simulink model "ip"  (R2022b)
settings: Solver=FixedStepAuto  StartTime=0.0  StopTime=inf  FixedStep=Ts  RelTol=1e-3
values from neighbouring files (symbols this model uses):
  kLqr = [-58.3388321167 -3.68890430291 -0.316227766017 -0.543428779836 0.0629976019045]    [K_lqr.mat]    (also in calculate_lqr.m = lqr(A, B, Q, RLQR))
undefined symbols (not defined in the file or in its folder): countsPerRev, currentGain, currentOffset, motorN, pendDwnValue
libraries: arduinolib x6, arduinosensorlib x1, hdlsllib x1
settings Model: SimulationMode=external  ExtModeTrigDuration=2  Creator=47954  LastModifiedBy=47954
settings SolverCC: AutoInsertRateTranBlk=on
settings OptimizationCC: EnhancedBackFolding=on  PassReuseOutputArgsThreshold=0  MaxStackSize=64  OptimizeBlockOrder=speed  DifferentSizesBufferReuse=on  OptimizationCustomize=off
settings DebuggingCC: ParameterPrecisionLossMsg=none  ParameterTunabilityLossMsg=error
settings HardwareCC: ProdBitPerInt=16  ProdBitPerPointer=16  ProdBitPerSizeT=16  ProdBitPerPtrDiffT=16  ProdLargestAtomicFloat=None  ProdWordSize=8  ProdLongLongMode=on  ProdHWDeviceType=Atmel->AVR  UseEmbeddedCoderFeatures=off  UseSimulinkCoderFeatures=off
settings ModelReferenceCC: EnableRefExpFcnMdlSchedulingChecks=on
settings SFSimCC: MATLABDynamicMemAlloc=off
settings RTWCC: Description=Embedded Coder  SystemTargetFile=ert.tlc  HardwareBoard=Arduino Mega 2560  TemplateMakefile=ert_default_tmf  RTWVerbose=off  Toolchain=Arduino AVR
settings CodeAppCC: ForceParamTrailComments=on  OperatorAnnotations=on  MangleLength=10
settings ERTTargetCC: ERTCustomFileBanners=off  SupportContinuousTime=on  SupportNonInlinedSFcns=on  RemoveResetFunc=off  SupportVariableSizeSignals=on  ModelStepFunctionPrototypeControlCompliant=off  ExtMode=on  ExtModeTransport=3  ExtModeStaticAlloc=on  ExtModeStaticAllocSize=2048  ExtModeMexFile=ext_xcp  ExtModeMexArgs=0 6 921600  ExtModeIntrfLevel=Level2 - Open  ERTSrcFileBannerTemplate=codertarget_code_template.cgt  ERTHdrFileBannerTemplate=codertarget_code_template.cgt  ERTDataSrcFileTemplate=codertarget_code_template.cgt  ERTDataHdrFileTemplate=codertarget_code_template.cgt

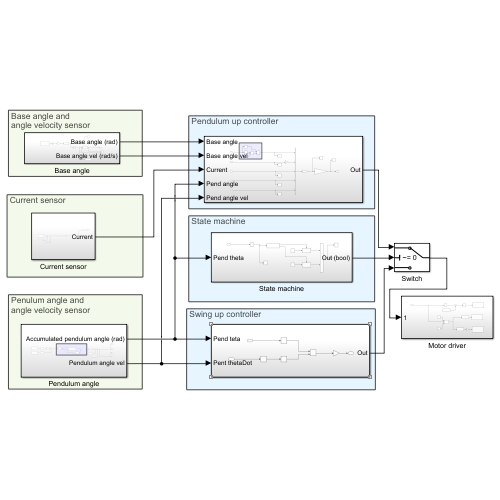
[thumbnail: Simulink's stored preview of the top-level diagram]
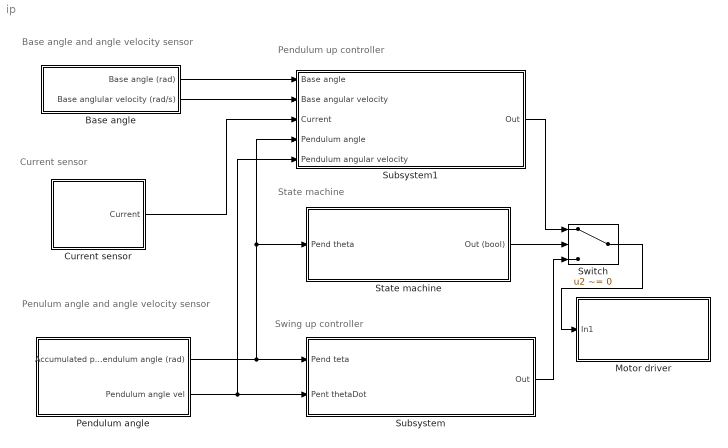
== system ip ==
  note: State machine
  note: Swing up controller
  note: Penulum angle and
      | angle velocity sensor
  note: Base angle and
      | angle velocity sensor
  note: Current sensor
  note: Pendulum up controller
  Base angle : Subsystem
  Current sensor : Subsystem
  Motor driver : Subsystem
  Pendulum angle : Subsystem
  State machine : Subsystem
  Subsystem : Subsystem
  Subsystem1 : Subsystem
  Switch : Switch  Criteria=u2 ~= 0  SaturateOnIntegerOverflow=off  InputSameDT=off
  wires:
  Pendulum angle/1(Accumulated pendulum angle (rad)) -> Subsystem1/4(Pendulum angle), State machine/1(Pend theta), Subsystem/1(Pend teta)
  State machine/1(Out (bool)) -> Switch/2
  Subsystem/1(Out) -> Switch/3
  Pendulum angle/2(Pendulum angle vel) -> Subsystem/2(Pent thetaDot), Subsystem1/5(Pendulum angular velocity)
  Subsystem1/1(Out) -> Switch/1
  Base angle/1(Base angle (rad)) -> Subsystem1/1(Base angle)
  Base angle/2(Base anglular velocity (rad/s)) -> Subsystem1/2(Base angular velocity)
  Switch/1 -> Motor driver/1(In1)
  Current sensor/1(Current) -> Subsystem1/3(Current)

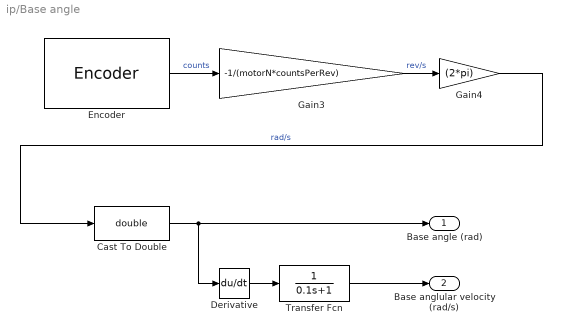
== system ip/Base angle ==
  Cast To Double : DataTypeConversion  OutDataTypeStr=double  SaturateOnIntegerOverflow=off  RndMeth=Floor
  Derivative : Derivative
  Encoder : arduinosensorlib/Encoder  InputA=2  InputB=3  Mode=No reset  SampleTime=-1
  Gain3 : Gain  Gain=-1/(motorN*countsPerRev)
  Gain4 : Gain  Gain=(2*pi)
  Transfer Fcn : TransferFcn  Denominator=[0.1 1]
  Base angle (rad) : Outport
  Base anglular velocity (rad/s) : Outport  Port=2
  wires:
  Gain3/1 -> Gain4/1  "rev/s"
  Gain4/1 -> Cast To Double/1  "rad/s"
  Encoder/1 -> Gain3/1  "counts"
  Transfer Fcn/1 -> Base anglular velocity (rad/s)/1
  Derivative/1 -> Transfer Fcn/1
  Cast To Double/1 -> Base angle (rad)/1, Derivative/1

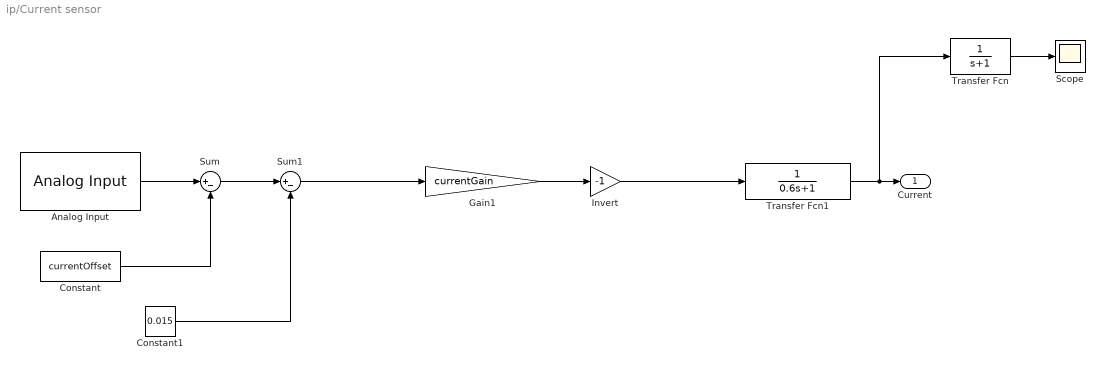
== system ip/Current sensor ==
  Analog Input : arduinolib/Analog Input  pinNumber=10  ReadResultsOnly=off  ConversionTriggerSource=Software  ExternalTriggerType=uint32( 0 )  OutputDataType=uint16  EnableConversionCompleteNotify=off  EnableOuputStatus=off  SampleTime=-1  blockPlatform=arduino
  Constant : Constant  Value=currentOffset
  Constant1 : Constant  Value=0.015
  Gain1 : Gain  Gain=currentGain
  Invert : Gain  Gain=-1
  Scope : Scope
  Sum : Sum  Inputs=|+-
  Sum1 : Sum  Inputs=|+-
  Transfer Fcn : TransferFcn  Denominator=[1 1]
  Transfer Fcn1 : TransferFcn  Denominator=[0.6 1]
  Current : Outport
  wires:
  Constant/1 -> Sum/2
  Analog Input/1 -> Sum/1
  Invert/1 -> Transfer Fcn1/1
  Sum/1 -> Sum1/1
  Gain1/1 -> Invert/1
  Transfer Fcn1/1 -> Transfer Fcn/1, Current/1
  Transfer Fcn/1 -> Scope/1
  Sum1/1 -> Gain1/1
  Constant1/1 -> Sum1/2

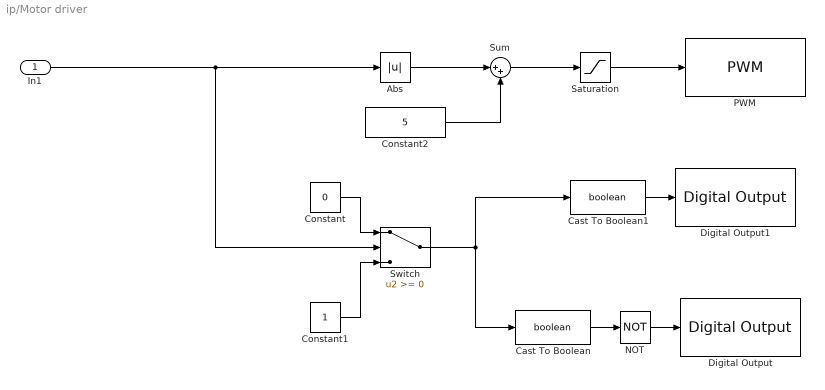
== system ip/Motor driver ==
  In1 : Inport
  Abs : Abs  SaturateOnIntegerOverflow=off
  Cast To Boolean : DataTypeConversion  OutDataTypeStr=boolean  SaturateOnIntegerOverflow=off  RndMeth=Floor
  Cast To Boolean1 : DataTypeConversion  OutDataTypeStr=boolean  SaturateOnIntegerOverflow=off  RndMeth=Floor
  Constant : Constant  Value=0
  Constant1 : Constant
  Constant2 : Constant  Value=5
  Digital Output : arduinolib/Digital Output  pinNumber=4  Direction=output  blockPlatform=arduino
  Digital Output1 : arduinolib/Digital Output  pinNumber=5  Direction=output  blockPlatform=arduino
  NOT : Logic  Operator=NOT  IconShape=distinctive  AllPortsSameDT=off  OutDataTypeStr=boolean
  PWM : arduinolib/PWM  pinNumber=13  frequencyType=Specify  desiredFrequency=490.2*2  achievableFrequency=980.4
  Saturation : Saturate  UpperLimit=255  LowerLimit=-255
  Sum : Sum  Inputs=|++
  Switch : Switch  SaturateOnIntegerOverflow=off  InputSameDT=off
  wires:
  Constant1/1 -> Switch/3
  Cast To Boolean1/1 -> Digital Output1/1
  Constant/1 -> Switch/1
  Constant2/1 -> Sum/2
  In1/1 -> Abs/1, Switch/2
  Switch/1 -> Cast To Boolean/1, Cast To Boolean1/1
  Cast To Boolean/1 -> NOT/1
  NOT/1 -> Digital Output/1
  Abs/1 -> Sum/1
  Sum/1 -> Saturation/1
  Saturation/1 -> PWM/1

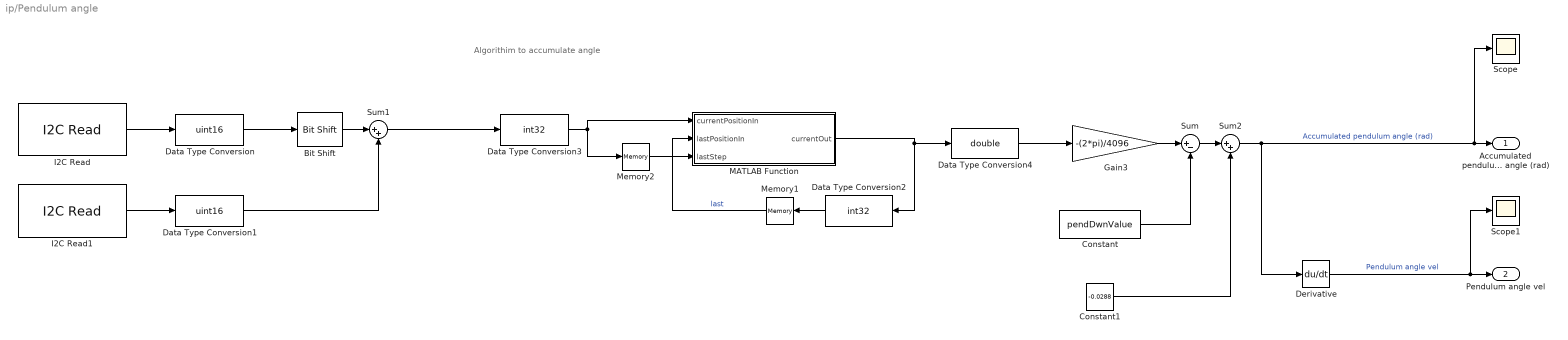
== system ip/Pendulum angle ==
  note: Algorithim to accumulate angle
  Bit Shift : hdlsllib/Logic and Bit Operations/Bit Shift  mode=Shift Left Logical  N=8
  Constant : Constant  Value=pendDwnValue
  Constant1 : Constant  Value=-0.0288
  Data Type Conversion : DataTypeConversion  OutDataTypeStr=uint16  SaturateOnIntegerOverflow=off  RndMeth=Floor
  Data Type Conversion1 : DataTypeConversion  OutDataTypeStr=uint16  SaturateOnIntegerOverflow=off  RndMeth=Floor
  Data Type Conversion2 : DataTypeConversion  OutDataTypeStr=int32  SaturateOnIntegerOverflow=off  RndMeth=Floor
  Data Type Conversion3 : DataTypeConversion  OutDataTypeStr=int32  SaturateOnIntegerOverflow=off  RndMeth=Floor
  Data Type Conversion4 : DataTypeConversion  OutDataTypeStr=double  SaturateOnIntegerOverflow=off  RndMeth=Floor
  Derivative : Derivative
  Gain3 : Gain  Gain=-(2*pi)/4096
  I2C Read : arduinolib/I2C Read  I2CModule=0  Mode=Master  SlaveAddress=0x36  SlaveByteOrder=BigEndian  Direction=Receiver  RegisterAddressMode=on  RegisterAddress=0x0c  SlaveDataType=uint8  DataLength=1  NoAck=off  RepeatedStart=off  OutputStatus=off  blockPlatform=ARDUINO  SampleTime=-1
  I2C Read1 : arduinolib/I2C Read  I2CModule=0  Mode=Master  SlaveAddress=0x36  SlaveByteOrder=BigEndian  Direction=Receiver  RegisterAddressMode=on  RegisterAddress=0x0d  SlaveDataType=uint8  DataLength=1  NoAck=off  RepeatedStart=off  OutputStatus=off  blockPlatform=ARDUINO  SampleTime=-1
  MATLAB Function : MATLAB Function  TreatAsAtomicUnit=on
  Memory1 : Memory
  Memory2 : Memory
  Scope : Scope
  Scope1 : Scope
  Sum : Sum  Inputs=|+-
  Sum1 : Sum  Inputs=|++
  Sum2 : Sum  Inputs=|++
  Accumulated pendulum angle (rad) : Outport
  Pendulum angle vel : Outport  Port=2
  wires:
  Memory2/1 -> MATLAB Function/3(lastStep)
  I2C Read/1 -> Data Type Conversion/1
  Data Type Conversion3/1 -> Memory2/1, MATLAB Function/1(currentPositionIn)
  Sum1/1 -> Data Type Conversion3/1
  I2C Read1/1 -> Data Type Conversion1/1
  Bit Shift/1 -> Sum1/1
  Memory1/1 -> MATLAB Function/2(lastPositionIn)  "last"
  Data Type Conversion1/1 -> Sum1/2
  Data Type Conversion/1 -> Bit Shift/1
  MATLAB Function/1(currentOut) -> Data Type Conversion2/1, Data Type Conversion4/1
  Data Type Conversion2/1 -> Memory1/1
  Data Type Conversion4/1 -> Gain3/1
  Gain3/1 -> Sum/1
  Constant/1 -> Sum/2
  Sum2/1 -> Accumulated pendulum angle (rad)/1, Scope/1, Derivative/1  "Accumulated pendulum angle (rad)"
  Sum/1 -> Sum2/1
  Constant1/1 -> Sum2/2
  Derivative/1 -> Scope1/1, Pendulum angle vel/1  "Pendulum angle vel"

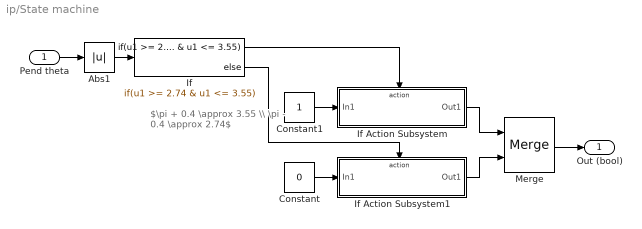
== system ip/State machine ==
  note: $\pi + 0.4 \approx 3.55 \\ \pi - 0.4 \approx 2.74$
  Pend theta : Inport
  Abs1 : Abs  SaturateOnIntegerOverflow=off
  Constant : Constant  Value=0
  Constant1 : Constant
  If : If  IfExpression=u1 >= 2.74 & u1 <= 3.55
  If Action Subsystem : Subsystem  TreatAsAtomicUnit=on
  If Action Subsystem1 : Subsystem  TreatAsAtomicUnit=on
  Merge : Merge
  Out (bool) : Outport
  wires:
  Constant1/1 -> If Action Subsystem/1(In1)
  If Action Subsystem/1(Out1) -> Merge/1
  If/1 -> If Action Subsystem/Action
  Pend theta/1 -> Abs1/1
  Merge/1 -> Out (bool)/1
  If/2 -> If Action Subsystem1/Action
  If Action Subsystem1/1(Out1) -> Merge/2
  Constant/1 -> If Action Subsystem1/1(In1)
  Abs1/1 -> If/1

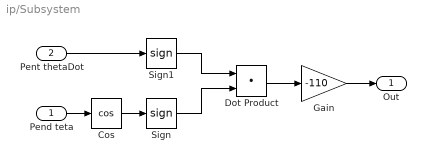
== system ip/Subsystem ==
  Pend teta : Inport
  Pent thetaDot : Inport  Port=2
  Cos : Trigonometry  Operator=cos
  Dot Product : DotProduct  OutDataTypeStr=Inherit: Inherit via internal rule
  Gain : Gain  Gain=-110
  Sign : Signum
  Sign1 : Signum
  Out : Outport
  wires:
  Pend teta/1 -> Cos/1
  Sign1/1 -> Dot Product/1
  Pent thetaDot/1 -> Sign1/1
  Dot Product/1 -> Gain/1
  Sign/1 -> Dot Product/2
  Cos/1 -> Sign/1
  Gain/1 -> Out/1

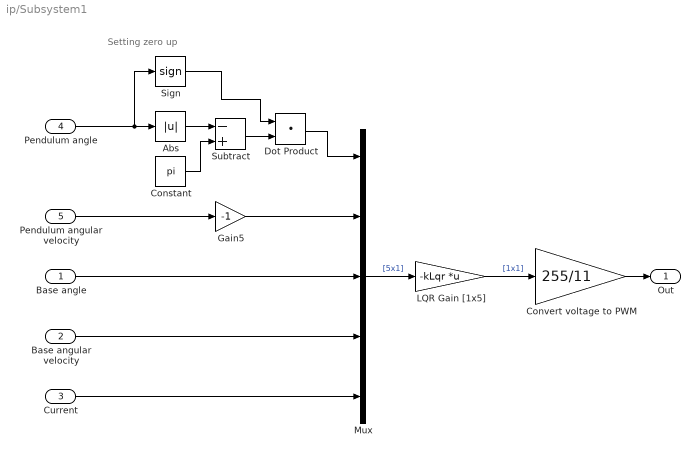
== system ip/Subsystem1 ==
  note: Setting zero up
  Base angle : Inport
  Base angular velocity : Inport  Port=2
  Current : Inport  Port=3
  Pendulum angle : Inport  Port=4
  Pendulum angular velocity : Inport  Port=5
  Abs : Abs  SaturateOnIntegerOverflow=off
  Constant : Constant  Value=pi
  Convert voltage to PWM : Gain  Gain=255/11
  Dot Product : DotProduct  OutDataTypeStr=Inherit: Inherit via internal rule
  Gain5 : Gain  Gain=-1
  LQR Gain [1x5] : Gain  Gain=-kLqr  Multiplication=Matrix(K*u)
  Mux : Mux  Inputs=5
  Sign : Signum
  Subtract : Sum  Inputs=-+
  Out : Outport
  wires:
  Pendulum angle/1 -> Sign/1, Abs/1
  Abs/1 -> Subtract/1
  Constant/1 -> Subtract/2
  Subtract/1 -> Dot Product/2
  Sign/1 -> Dot Product/1
  Dot Product/1 -> Mux/1
  Pendulum angular velocity/1 -> Gain5/1
  Base angle/1 -> Mux/3
  Base angular velocity/1 -> Mux/4
  Current/1 -> Mux/5
  Mux/1 -> LQR Gain [1x5]/1  "[5x1]"
  LQR Gain [1x5]/1 -> Convert voltage to PWM/1  "[1x1]"
  Convert voltage to PWM/1 -> Out/1
  Gain5/1 -> Mux/2

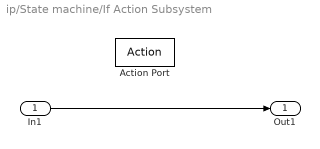
== system ip/State machine/If Action Subsystem ==
  In1 : Inport
  Action Port : ActionPort  ActionPortLabel=if(u1 >= 2.74 & u1 <= 3.55)
  Out1 : Outport
  wires:
  In1/1 -> Out1/1

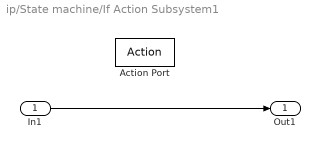
== system ip/State machine/If Action Subsystem1 ==
  In1 : Inport
  Action Port : ActionPort  ActionPortLabel=else
  Out1 : Outport
  wires:
  In1/1 -> Out1/1

== matlab function ip/Pendulum angle/MATLAB Function ==
  data: currentPositionIn input; currentOut output; lastPositionIn input; lastStep input
function currentOut  = fcn(currentPositionIn, lastPositionIn, lastStep)

% currentPositionIn = value
% lastPositionIn = _position
% lastStep = _lastPosition


%  whole rotation CW?
if((lastStep > 2048) && (currentPositionIn <(lastStep - 2048)))
    currentOut = lastPositionIn + 4096 - lastStep + currentPositionIn;
elseif((currentPositionIn > 2048) && ( lastStep < (currentPositionIn - 2048)))
    currentOut = lastPositionIn - 4096 - lastStep + currentPositionIn;
else
    currentOut = lastPositionIn - lastStep + currentPositionIn;
end
